simulink model "Ex6"  (R2020a)
settings: Solver=VariableStepAuto  StartTime=0.0  StopTime=10.0  RelTol=1e-3
settings Model: Creator=Joao Loureiro  LastModifiedBy=Joao Loureiro

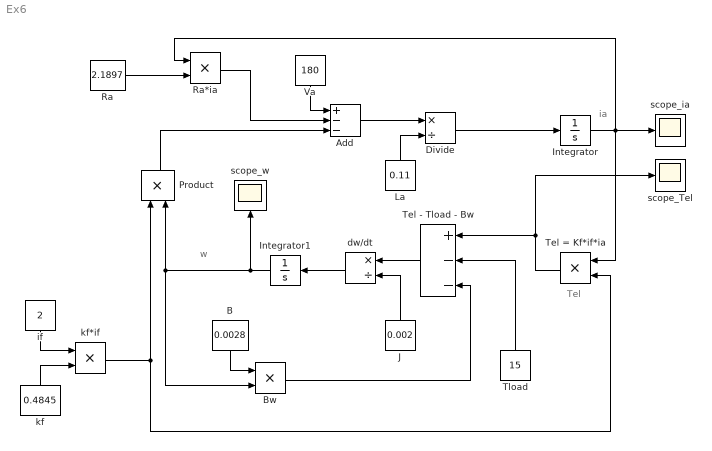
== system Ex6 ==
  note: ia
  note: w
  note: Tel
  Add : Sum  Inputs=+--
  B : Constant  Value=0.0028
  Bw : Product
  Divide : Product  Inputs=*/
  Integrator : Integrator
  Integrator1 : Integrator
  J : Constant  Value=0.002
  La : Constant  Value=0.11
  Product : Product
  Ra : Constant  Value=2.1897
  Ra*ia : Product
  Tel - Tload - Bw : Sum  Inputs=+--
  Tel = Kf*if*ia : Product
  Tload : Constant  Value=15
  Va : Constant  Value=180
  dw/dt : Product  Inputs=*/
  if : Constant  Value=2
  kf : Constant  Value=0.4845
  kf*if : Product
  scope_Tel : Scope
  scope_ia : Scope
  scope_w : Scope
  wires:
  Ra/1 -> Ra*ia/2
  La/1 -> Divide/2
  Tel - Tload - Bw/1 -> dw/dt/1
  Integrator1/1 -> Bw/2, Product/2, scope_w/1
  Tel = Kf*if*ia/1 -> Tel - Tload - Bw/1, scope_Tel/1
  Bw/1 -> Tel - Tload - Bw/3
  Va/1 -> Add/1
  B/1 -> Bw/1
  Integrator/1 -> scope_ia/1, Tel = Kf*if*ia/1, Ra*ia/1
  Add/1 -> Divide/1
  Product/1 -> Add/3
  dw/dt/1 -> Integrator1/1
  Ra*ia/1 -> Add/2
  kf*if/1 -> Product/1, Tel = Kf*if*ia/2
  Divide/1 -> Integrator/1
  if/1 -> kf*if/1
  kf/1 -> kf*if/2
  J/1 -> dw/dt/2
  Tload/1 -> Tel - Tload - Bw/2
